simulink model "OrientationTest"  (R2015a)
settings: Solver=ode45  StartTime=0.0  StopTime=50.0  RelTol=1e-5
libraries: aerolibutil x4
settings Model: Creator=mangerer  LastModifiedBy=mangerer

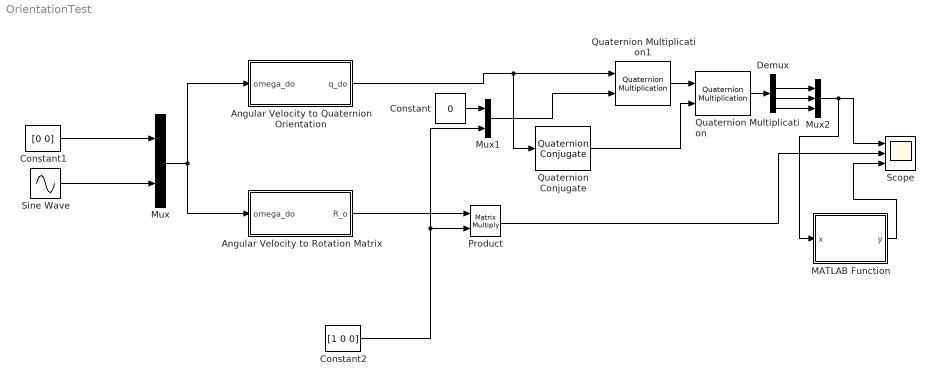
== system OrientationTest ==
  Angular Velocity to Quaternion Orientation : Subsystem
  Angular Velocity to Rotation Matrix : Subsystem
  Constant : Constant  Value=0
  Constant1 : Constant  Value=[0 0]
  Constant2 : Constant  Value=[1 0 0]
  Demux : Demux
  MATLAB Function : MATLAB Function  TreatAsAtomicUnit=on
  Mux : Mux  Inputs=2
  Mux1 : Mux  Inputs=2
  Mux2 : Mux  Inputs=3
  Product : Product  Multiplication=Matrix(*)
  Quaternion Conjugate : aerolibutil/Quaternion Conjugate
  Quaternion Multiplication : aerolibutil/Quaternion Multiplication
  Quaternion Multiplication1 : aerolibutil/Quaternion Multiplication
  Scope : Scope  NumInputPorts=3
      settings: ShowLegends=on  YMin=-5~-5~-5  YMax=5~5~5
  Sine Wave : Sin  Frequency=0.5*pi  SampleTime=0
  wires:
  Constant1/1 -> Mux/1
  Constant/1 -> Mux1/1
  Quaternion Multiplication/1 -> Demux/1
  Constant2/1 -> Product/2, Mux1/2
  Angular Velocity to Rotation Matrix/1(R_o) -> Product/1
  Product/1 -> Scope/2
  Demux/4 -> Mux2/3
  Demux/3 -> Mux2/2
  Demux/2 -> Mux2/1
  Mux2/1 -> MATLAB Function/1(x), Scope/1
  Mux/1 -> Angular Velocity to Quaternion Orientation/1(omega_do), Angular Velocity to Rotation Matrix/1(omega_do)
  Sine Wave/1 -> Mux/2
  Quaternion Multiplication1/1 -> Quaternion Multiplication/1
  Angular Velocity to Quaternion Orientation/1(q_do) -> Quaternion Conjugate/1, Quaternion Multiplication1/1
  Mux1/1 -> Quaternion Multiplication1/2
  Quaternion Conjugate/1 -> Quaternion Multiplication/2
  MATLAB Function/1(y) -> Scope/3

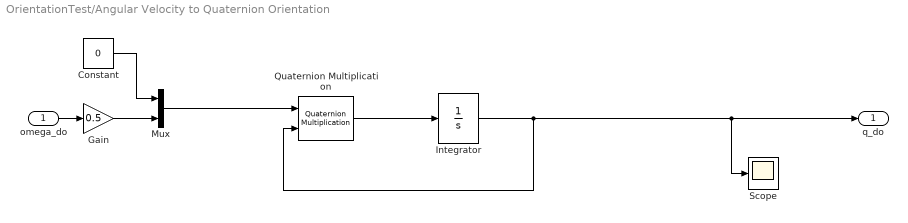
== system OrientationTest/Angular Velocity to Quaternion Orientation ==
  omega_do : Inport
  Constant : Constant  Value=0
  Gain : Gain  Gain=0.5
  Integrator : Integrator  InitialCondition=[1; 0; 0; 0]
  Mux : Mux  Inputs=2
  Quaternion Multiplication : aerolibutil/Quaternion Multiplication
  Scope : Scope
      settings: ShowLegends=on  SaveName=ScopeData9
  q_do : Outport
  wires:
  omega_do/1 -> Gain/1
  Gain/1 -> Mux/2
  Constant/1 -> Mux/1
  Quaternion Multiplication/1 -> Integrator/1
  Integrator/1 -> Quaternion Multiplication/2, Scope/1, q_do/1
  Mux/1 -> Quaternion Multiplication/1

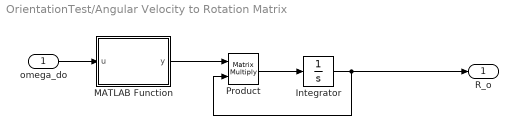
== system OrientationTest/Angular Velocity to Rotation Matrix ==
  omega_do : Inport
  Integrator : Integrator  InitialCondition=[1 0 0; 0 1 0; 0 0 1]
  MATLAB Function : MATLAB Function  TreatAsAtomicUnit=on
  Product : Product  Multiplication=Matrix(*)
  R_o : Outport
  wires:
  Product/1 -> Integrator/1
  Integrator/1 -> R_o/1, Product/2
  omega_do/1 -> MATLAB Function/1(u)
  MATLAB Function/1(y) -> Product/1

== matlab function OrientationTest/MATLAB Function ==
  data: x input; y output
function y = abs(x)
%#codegen

y = x(1)^2 + x(2)^2 + x(3)^2;

== matlab function OrientationTest/Angular Velocity to Rotation Matrix/MATLAB Function ==
  data: u input; y output
function y = Skew(u)
y = skew_sm(u)
